simulink model "DT_enviroment_state_machine"  (R2024b)
settings: Solver=FixedStepAuto  StartTime=0.0  StopTime=120  FixedStep=1e-3  RelTol=1e-3
InitFcn:
  | V_bias_cmd=0;
  | enable_cmd=0;
  | mode_cmd=0;
  | P_batt_cmd=0;
libraries: fl_lib x14, nesl_utility x12, batteryecm_lib x2, eeGeneralControl x2, slpidlib x2, simulink x1, spspowerguiLib x1
(part 2 of 2)

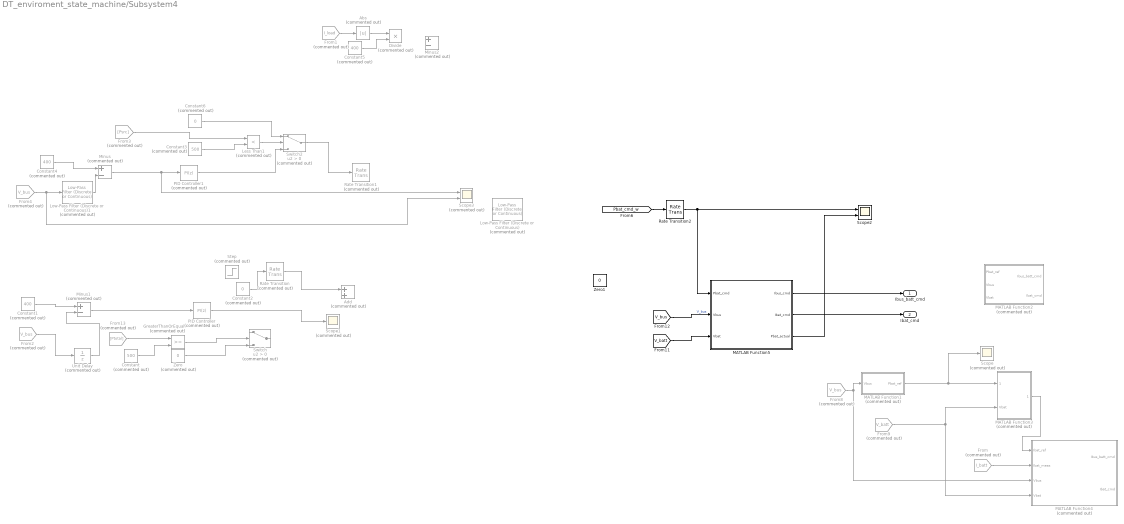
== system DT_enviroment_state_machine/Subsystem4 ==
  Abs : Abs  Commented=on  SaturateOnIntegerOverflow=off
  Add : Sum  Commented=on
  Constant : Constant  Commented=on  Value=500  SampleTime=-1
  Constant1 : Constant  Commented=on  Value=400
  Constant2 : Constant  Commented=on  Value=0  SampleTime=-1
  Constant3 : Constant  Commented=on  Value=500
  Constant4 : Constant  Commented=on  Value=400
  Constant5 : Constant  Commented=on  Value=400
  Constant6 : Constant  Commented=on  Value=0
  Divide : Product  Commented=on  Inputs=**
  From : From  Commented=on  GotoTag=I_batt  TagVisibility=global
  From1 : From  Commented=on  GotoTag=I_load  TagVisibility=global
  From13 : From  Commented=on  GotoTag=Ptotal  TagVisibility=global
  From2 : From  Commented=on  GotoTag=V_bus  TagVisibility=global
  From3 : From  Commented=on  GotoTag=Psrc  TagVisibility=global
  From4 : From  Commented=on  GotoTag=V_bus  TagVisibility=global
  From8 : From  Commented=on  GotoTag=V_bus  TagVisibility=global
  From9 : From  Commented=on  GotoTag=V_batt  TagVisibility=global
  GreaterThanOrEqual : RelationalOperator  Commented=on  OutDataTypeStr=boolean  RndMeth=Simplest  InputSameDT=off
  Less Than1 : RelationalOperator  Commented=on  Operator=<  OutDataTypeStr=boolean  RndMeth=Simplest  InputSameDT=off
  Low-Pass Filter (Discrete or Continuous) : eeGeneralControl/Low-Pass Filter (Discrete or Continuous)  Commented=on  K=1  T=50000/1000  B=inf  A=-inf  init_option=Inherited from block input  x0=0  Ts=-1
  Low-Pass Filter (Discrete or Continuous)1 : eeGeneralControl/Low-Pass Filter (Discrete or Continuous)  Commented=on  K=1  T=50000/1000  B=inf  A=-inf  init_option=Inherited from block input  x0=0  Ts=-1
  MATLAB Function1 : MATLAB Function  Commented=on  TreatAsAtomicUnit=on
  MATLAB Function2 : MATLAB Function  Commented=on  TreatAsAtomicUnit=on
  MATLAB Function3 : MATLAB Function  Commented=on  TreatAsAtomicUnit=on
  MATLAB Function4 : MATLAB Function  Commented=on  TreatAsAtomicUnit=on
  MATLAB Function5 : MATLAB Function  TreatAsAtomicUnit=on
  Minus : Sum  Commented=on  Inputs=+-
  Minus1 : Sum  Commented=on  Inputs=+-
  Minus2 : Sum  Commented=on  Inputs=+-
  PID Controller : slpidlib/PID Controller  Commented=on  Controller=PI  Form=Parallel  TimeDomain=Discrete-time  UseExternalTs=off  SampleTime=-1  IntegratorMethod=Forward Euler  FilterMethod=Forward Euler  ControllerParametersSource=internal  P=0.5  I=1  UseKiTs=off  D=0  UseExternalDerivativeSource=off  N=100  UseFilter=on  TunerSelectOption=Transfer Function Based (PID Tuner App)  InitialConditionSource=internal  InitialConditionForIntegrator=0  InitialConditionForFilter=0  DifferentiatorICPrevScaledInput=0  ExternalReset=none  TrackingMode=off  Kt=1  LimitOutput=off  SatLimitsSource=internal  UpperSaturationLimit=inf  LowerSaturationLimit=-inf  LinearizeAsGain=on  AntiWindupMode=clamping  Kb=1  LimitIntegrator=off  UpperIntegratorSaturationLimit=inf  LowerIntegratorSaturationLimit=-inf  POutMin=[]  POutMax=[]  IOutMin=[]  IOutMax=[]  DOutMin=[]  DOutMax=[]  NOutMin=[]  NOutMax=[]  SumOutMin=[]  SumOutMax=[]  SaturationOutMin=[]  SaturationOutMax=[]  PParamMin=[]  PParamMax=[]  IParamMin=[]  IParamMax=[]  DParamMin=[]  DParamMax=[]  NParamMin=[]  NParamMax=[]  KbParamMin=[]  KbParamMax=[]  KtParamMin=[]  KtParamMax=[]  KbOutMin=[]  KbOutMax=[]  KtOutMin=[]  KtOutMax=[]  IntegratorOutMin=[]  IntegratorOutMax=[]  FilterOutMin=[]  FilterOutMax=[]  SumI1OutMin=[]  SumI1OutMax=[]  SumI2OutMin=[]  SumI2OutMax=[]  SumI3OutMin=[]  SumI3OutMax=[]  SumI4OutMin=[]  SumI4OutMax=[]  SumDOutMin=[]  SumDOutMax=[]  DifferentiatorOutMin=[]  DifferentiatorOutMax=[]  FilterDiffOutCoefMin=[]  FilterDiffOutCoefMax=[]  ReciprocalOutMin=[]  ReciprocalOutMax=[]  SumDenOutMin=[]  SumDenOutMax=[]  SumNumOutMin=[]  SumNumOutMax=[]  DivideOutMin=[]  DivideOutMax=[]  UdiffTsProdOutMin=[]  UdiffTsProdOutMax=[]  NTsProdOutMin=[]  NTsProdOutMax=[]  UintegralTsProdOutMin=[]  UintegralTsProdOutMax=[]  UngainTsProdOutMin=[]  UngainTsProdOutMax=[]  ClampingZeroOutDataTypeStr=Inherit: Inherit via back propagation  ClampingZeroOutMin=[]  ClampingZeroOutMax=[]  FilterDenConstantOutDataTypeStr=Inherit: Inherit via back propagation  FilterDenConstantOutMin=[]  FilterDenConstantOutMax=[]  PCopyOutDataTypeStr=Inherit: Inherit via back propagation  PCopyOutMin=[]  PCopyOutMax=[]  NCopyOutDataTypeStr=Inherit: Inherit via back propagation  NCopyOutMin=[]  NCopyOutMax=[]  IntegratorContinuousStateAttributes=''  IntegratorStateMustResolveToSignalObject=off  IntegratorRTWStateStorageClass=Auto  FilterContinuousStateAttributes=''  FilterStateMustResolveToSignalObject=off  FilterRTWStateStorageClass=Auto  ParallelPVariant=InternalParameters  IdealPVariant=Disabled  IVariant=InternalParameters  DVariant=Disabled  IntegratorVariant=Discrete  SatVariant=Disabled  AWVariant=Passthrough  PCopyVariant=Disabled  TRVariant=Disabled  FdbkBlocksVariant=Forward  IdealPFdbkVariant=Disabled  SatFdbkVariant=Disabled  DerivativeFilterVariant=Disabled  NVariant=Disabled  NCopyVariant=Disabled_SignalSpec  FilterICVariant=Disabled  IntegratorICVariant=InternalICs  ExternalResetVariant=Disabled  TRSumVariant=Passthrough  SumFdbkVariant=Disabled  SumVariant=Sum_PI  TsampFilterVariant=InternalTs  TsampNgainVariant=Passthrough  TsampIntegralVariant=Disabled_SignalSpec  ExternalSaturationOutDataTypeStr=Inherit: Same as second input  DerivativeSourceVariant=Disabled  PreIntVariant=InternalPreInt
  PID Controller1 : slpidlib/PID Controller  Commented=on  Controller=PI  Form=Parallel  TimeDomain=Discrete-time  UseExternalTs=off  SampleTime=-1  IntegratorMethod=Forward Euler  FilterMethod=Forward Euler  ControllerParametersSource=internal  P=0.01  I=1  UseKiTs=off  D=0  UseExternalDerivativeSource=off  N=100  UseFilter=on  TunerSelectOption=Transfer Function Based (PID Tuner App)  InitialConditionSource=internal  InitialConditionForIntegrator=0  InitialConditionForFilter=0  DifferentiatorICPrevScaledInput=0  ExternalReset=none  TrackingMode=off  Kt=1  LimitOutput=on  SatLimitsSource=internal  UpperSaturationLimit=1000  LowerSaturationLimit=-1000  LinearizeAsGain=on  AntiWindupMode=none  Kb=1  LimitIntegrator=off  UpperIntegratorSaturationLimit=inf  LowerIntegratorSaturationLimit=-inf  POutMin=[]  POutMax=[]  IOutMin=[]  IOutMax=[]  DOutMin=[]  DOutMax=[]  NOutMin=[]  NOutMax=[]  SumOutMin=[]  SumOutMax=[]  SaturationOutMin=[]  SaturationOutMax=[]  PParamMin=[]  PParamMax=[]  IParamMin=[]  IParamMax=[]  DParamMin=[]  DParamMax=[]  NParamMin=[]  NParamMax=[]  KbParamMin=[]  KbParamMax=[]  KtParamMin=[]  KtParamMax=[]  KbOutMin=[]  KbOutMax=[]  KtOutMin=[]  KtOutMax=[]  IntegratorOutMin=[]  IntegratorOutMax=[]  FilterOutMin=[]  FilterOutMax=[]  SumI1OutMin=[]  SumI1OutMax=[]  SumI2OutMin=[]  SumI2OutMax=[]  SumI3OutMin=[]  SumI3OutMax=[]  SumI4OutMin=[]  SumI4OutMax=[]  SumDOutMin=[]  SumDOutMax=[]  DifferentiatorOutMin=[]  DifferentiatorOutMax=[]  FilterDiffOutCoefMin=[]  FilterDiffOutCoefMax=[]  ReciprocalOutMin=[]  ReciprocalOutMax=[]  SumDenOutMin=[]  SumDenOutMax=[]  SumNumOutMin=[]  SumNumOutMax=[]  DivideOutMin=[]  DivideOutMax=[]  UdiffTsProdOutMin=[]  UdiffTsProdOutMax=[]  NTsProdOutMin=[]  NTsProdOutMax=[]  UintegralTsProdOutMin=[]  UintegralTsProdOutMax=[]  UngainTsProdOutMin=[]  UngainTsProdOutMax=[]  ClampingZeroOutDataTypeStr=Inherit: Inherit via back propagation  ClampingZeroOutMin=[]  ClampingZeroOutMax=[]  FilterDenConstantOutDataTypeStr=Inherit: Inherit via back propagation  FilterDenConstantOutMin=[]  FilterDenConstantOutMax=[]  PCopyOutDataTypeStr=Inherit: Inherit via back propagation  PCopyOutMin=[]  PCopyOutMax=[]  NCopyOutDataTypeStr=Inherit: Inherit via back propagation  NCopyOutMin=[]  NCopyOutMax=[]  IntegratorContinuousStateAttributes=''  IntegratorStateMustResolveToSignalObject=off  IntegratorRTWStateStorageClass=Auto  FilterContinuousStateAttributes=''  FilterStateMustResolveToSignalObject=off  FilterRTWStateStorageClass=Auto  ParallelPVariant=InternalParameters  IdealPVariant=Disabled  IVariant=InternalParameters  DVariant=Disabled  IntegratorVariant=Discrete  SatVariant=Enabled  AWVariant=Passthrough  PCopyVariant=Disabled  TRVariant=Disabled  FdbkBlocksVariant=Forward  IdealPFdbkVariant=Disabled  SatFdbkVariant=Disabled  DerivativeFilterVariant=Disabled  NVariant=Disabled  NCopyVariant=Disabled_SignalSpec  FilterICVariant=Disabled  IntegratorICVariant=InternalICs  ExternalResetVariant=Disabled  TRSumVariant=Passthrough  SumFdbkVariant=Disabled  SumVariant=Sum_PI  TsampFilterVariant=InternalTs  TsampNgainVariant=Passthrough  TsampIntegralVariant=Disabled_SignalSpec  ExternalSaturationOutDataTypeStr=Inherit: Same as second input  DerivativeSourceVariant=Disabled  PreIntVariant=InternalPreInt
  Rate Transition : RateTransition  Commented=on
  Rate Transition1 : RateTransition  Commented=on
  Rate Transition2 : RateTransition
  Scope : Scope  Commented=on
  Scope1 : Scope  Commented=on
  Scope2 : Scope  NumInputPorts=2
  Scope3 : Scope  Commented=on  NumInputPorts=2
  Step : Step  Commented=on  Time=170  After=-100  SampleTime=0
  Switch : Switch  Commented=on  Criteria=u2 > Threshold  SaturateOnIntegerOverflow=off  InputSameDT=off
  Switch2 : Switch  Commented=on  Criteria=u2 > Threshold  SaturateOnIntegerOverflow=off  InputSameDT=off
  Unit Delay : UnitDelay  Commented=on  SampleTime=-1  HasFrameUpgradeWarning=on
  Zero : Constant  Commented=on  Value=0  OutDataTypeStr=Inherit: Inherit via back propagation  SampleTime=-1
  Zero1 : Constant  Value=0  OutDataTypeStr=Inherit: Inherit via back propagation
  Ibus_batt_cmd : Outport
  Ibat_cmd : Outport  Port=2
  wires:
  From8/1 -> MATLAB Function4/3(Vbus), MATLAB Function1/1(Vbus)
  MATLAB Function5/1(Ibus_cmd) -> Ibus_batt_cmd/1
  MATLAB Function1/1(Pbat_ref) -> Scope/1, MATLAB Function3/1(Pbat_ref)
  From9/1 -> MATLAB Function3/2(Vbat), MATLAB Function4/4(Vbat)
  MATLAB Function3/1(Ibat_ref) -> MATLAB Function4/1(Ibat_ref)
  From/1 -> MATLAB Function4/2(Ibat_meas)
  MATLAB Function5/2(Ibat_cmd) -> Ibat_cmd/1
  [V_bus] -> MATLAB Function5/2(Vbus)  "V_bus"
  [V_batt] -> MATLAB Function5/3(Vbat)
  From13/1 -> GreaterThanOrEqual/1
  Constant/1 -> GreaterThanOrEqual/2
  GreaterThanOrEqual/1 -> Switch/2
  Zero/1 -> Switch/3
  ? -> Switch/1
  Unit Delay/1 -> Minus1/2
  Minus1/1 -> PID Controller/1
  Constant1/1 -> Minus1/1
  PID Controller/1 -> Scope1/1
  Rate Transition/1 -> Add/1
  Constant2/1 -> Rate Transition/1
  From2/1 -> Unit Delay/1
  From1/1 -> Abs/1
  Constant5/1 -> Divide/2
  From3/1 -> Less Than1/1
  Abs/1 -> Divide/1
  Constant3/1 -> Less Than1/2
  Less Than1/1 -> Switch2/2
  Constant6/1 -> Switch2/1
  Switch2/1 -> Rate Transition1/1
  MATLAB Function5/3(Pbat_actual) -> Scope2/2
  PID Controller1/1 -> Switch2/3
  Constant4/1 -> Minus/1
  From4/1 -> Scope3/2, Low-Pass Filter (Discrete or Continuous)1/1
  Minus/1 -> PID Controller1/1, Scope3/1
  Low-Pass Filter (Discrete or Continuous)1/1 -> Minus/2
  Rate Transition2/1 -> MATLAB Function5/1(Pbat_cmd), Scope2/1
  [Pbat_cmd_w] -> Rate Transition2/1

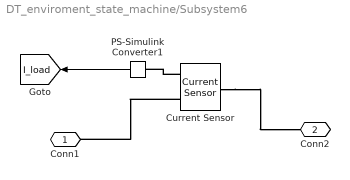
== system DT_enviroment_state_machine/Subsystem6 ==
  Current Sensor : fl_lib/Electrical/Electrical Sensors/Current Sensor
  PS-Simulink Converter1 : nesl_utility/PS-Simulink Converter  PhysicalDomain=network_engine_domain  SubClassName=ps_output  LeftPortType=input  RightPortType=output  PseudoPeriodic=off  Frequencies=[]  VectorFormat=inherit  Unit=inherit  AffineConversion=off
  Conn1 : PMIOPort  Side=Left
  Conn2 : PMIOPort  Port=2  Side=Right
  tag scope: I_load=global
  wires:
  PS-Simulink Converter1/1 -> [I_load]
  connections:
  Current Sensor/RConn1 -- PS-Simulink Converter1/LConn1
  Current Sensor/LConn1 -- Conn2/RConn1
  Current Sensor/RConn2 -- Conn1/RConn1

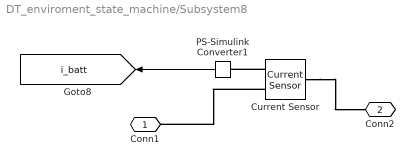
== system DT_enviroment_state_machine/Subsystem8 ==
  Current Sensor : fl_lib/Electrical/Electrical Sensors/Current Sensor
  PS-Simulink Converter1 : nesl_utility/PS-Simulink Converter  PhysicalDomain=network_engine_domain  SubClassName=ps_output  LeftPortType=input  RightPortType=output  PseudoPeriodic=off  Frequencies=[]  VectorFormat=inherit  Unit=inherit  AffineConversion=off
  Conn1 : PMIOPort  Side=Left
  Conn2 : PMIOPort  Port=2  Side=Right
  tag scope: i_batt=global
  wires:
  PS-Simulink Converter1/1 -> [i_batt]
  connections:
  Current Sensor/RConn1 -- PS-Simulink Converter1/LConn1
  Current Sensor/RConn2 -- Conn1/RConn1
  Current Sensor/LConn1 -- Conn2/RConn1

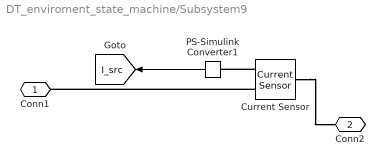
== system DT_enviroment_state_machine/Subsystem9 ==
  Current Sensor : fl_lib/Electrical/Electrical Sensors/Current Sensor
  PS-Simulink Converter1 : nesl_utility/PS-Simulink Converter  PhysicalDomain=network_engine_domain  SubClassName=ps_output  LeftPortType=input  RightPortType=output  PseudoPeriodic=off  Frequencies=[]  VectorFormat=inherit  Unit=inherit  AffineConversion=off
  Conn1 : PMIOPort  Side=Left
  Conn2 : PMIOPort  Port=2  Side=Right
  tag scope: I_src=global
  wires:
  PS-Simulink Converter1/1 -> [I_src]
  connections:
  Current Sensor/RConn1 -- PS-Simulink Converter1/LConn1
  Current Sensor/RConn2 -- Conn1/RConn1
  Current Sensor/LConn1 -- Conn2/RConn1

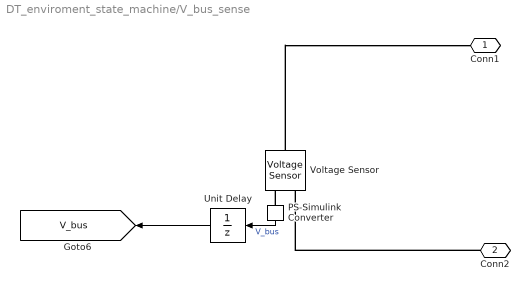
== system DT_enviroment_state_machine/V_bus_sense ==
  PS-Simulink Converter : nesl_utility/PS-Simulink Converter  PhysicalDomain=network_engine_domain  SubClassName=ps_output  LeftPortType=input  RightPortType=output  PseudoPeriodic=off  Frequencies=[]  VectorFormat=inherit  Unit=inherit  AffineConversion=off
  Unit Delay : UnitDelay  InitialCondition=400  SampleTime=-1  HasFrameUpgradeWarning=on
  Voltage Sensor : fl_lib/Electrical/Electrical Sensors/Voltage Sensor
  Conn1 : PMIOPort  Side=Left
  Conn2 : PMIOPort  Port=2  Side=Right
  tag scope: V_bus=global
  wires:
  PS-Simulink Converter/1 -> Unit Delay/1  "V_bus"
  Unit Delay/1 -> [V_bus]
  connections:
  PS-Simulink Converter/LConn1 -- Voltage Sensor/RConn1
  Conn2/RConn1 -- Voltage Sensor/RConn2
  Voltage Sensor/LConn1 -- Conn1/RConn1

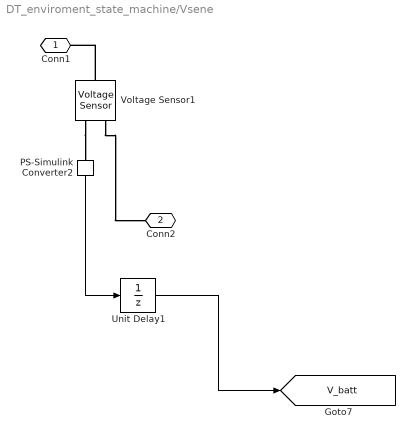
== system DT_enviroment_state_machine/Vsene ==
  PS-Simulink Converter2 : nesl_utility/PS-Simulink Converter  PhysicalDomain=network_engine_domain  SubClassName=ps_output  LeftPortType=input  RightPortType=output  PseudoPeriodic=off  Frequencies=[]  VectorFormat=inherit  Unit=inherit  AffineConversion=off
  Unit Delay1 : UnitDelay  InitialCondition=300  SampleTime=-1  HasFrameUpgradeWarning=on
  Voltage Sensor1 : fl_lib/Electrical/Electrical Sensors/Voltage Sensor
  Conn1 : PMIOPort  Side=Left
  Conn2 : PMIOPort  Port=2  Side=Right
  tag scope: V_batt=global
  wires:
  PS-Simulink Converter2/1 -> Unit Delay1/1
  Unit Delay1/1 -> [V_batt]
  connections:
  Voltage Sensor1/LConn1 -- Conn1/RConn1
  Voltage Sensor1/RConn1 -- PS-Simulink Converter2/LConn1
  Voltage Sensor1/RConn2 -- Conn2/RConn1

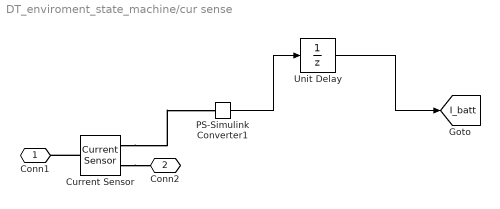
== system DT_enviroment_state_machine/cur sense ==
  Current Sensor : fl_lib/Electrical/Electrical Sensors/Current Sensor
  PS-Simulink Converter1 : nesl_utility/PS-Simulink Converter  PhysicalDomain=network_engine_domain  SubClassName=ps_output  LeftPortType=input  RightPortType=output  PseudoPeriodic=off  Frequencies=[]  VectorFormat=inherit  Unit=inherit  AffineConversion=off
  Unit Delay : UnitDelay  SampleTime=-1  HasFrameUpgradeWarning=on
  Conn1 : PMIOPort  Side=Left
  Conn2 : PMIOPort  Port=2  Side=Right
  tag scope: I_batt=global
  wires:
  PS-Simulink Converter1/1 -> Unit Delay/1
  Unit Delay/1 -> [I_batt]
  connections:
  Current Sensor/RConn1 -- PS-Simulink Converter1/LConn1
  Current Sensor/LConn1 -- Conn1/RConn1
  Current Sensor/RConn2 -- Conn2/RConn1

== matlab function DT_enviroment_state_machine/Subsystem4/MATLAB Function1 ==
  data: Vbus input; Pbat_ref output
% function Pbat_ref = battery_outer_bus_controller(Vbus)
% 
% % Positive Pbat_ref = battery discharges into the bus
% % Negative Pbat_ref = battery charges from the bus
% 
% Vref = 400;
% deadband = 2;
% 
% Pdis_max = 480;   % W, about 12 V * 40 A
% Pchg_max = 300;   % W, about 12 V * 25 A
% 
% Kp = 40;
% 
% err = Vref - Vbus;
% 
% if abs(err) < deadband
%     Pcmd = 0;
% else
%     Pcmd = Kp * err;
% end
% 
% Pbat_ref = min(max(Pcmd, -Pchg_max), Pdis_max);

function Pbat_ref = battery_outer_bus_controller(Vbus)

% Positive Pbat_ref = battery discharges into bus
% Negative Pbat_ref = battery charges from bus

Vref = 400;

Pdis_max = 480;   % W
Pchg_max = 300;   % W

Kp = 80;          % W/V
Ki = 300;         % W/(V*s)

Ts = 1e-3;        % match your controller sample time

persistent integ
if isempty(integ)
    integ = 0;
end

err = Vref - Vbus;

P_unsat = Kp*err + Ki*integ;

Pbat_ref = min(max(P_unsat, -Pchg_max), Pdis_max);

% Anti-windup
if Pbat_ref == P_unsat || ...
   (Pbat_ref == Pdis_max && err < 0) || ...
   (Pbat_ref == -Pchg_max && err > 0)
    integ = integ + err*Ts;
end

== matlab function DT_enviroment_state_machine/Subsystem1/MATLAB Function ==
  data: Isrc output; Vbus input
function Isrc = source_current_command(Vbus)

% 400 V regulated source with 500 W power limit

Vref = 400;
Pmax = 500;

Kp = 0.1;      % A/V
Ki = 5.0;      % A/(V*s)
Ts = 1e-3;     % match your controller sample time

persistent integ
if isempty(integ)
    integ = 0;
end

err = Vref - Vbus;

% Integrate only when bus is below/near reference
integ = integ + err * Ts;

Isrc_cmd = Kp*err + Ki*integ;

% Source cannot absorb current in this simple model
Isrc_cmd = max(Isrc_cmd, 0);

% Power limit
Vsafe = max(abs(Vbus), 100);
Isrc_pmax = Pmax / Vsafe;

% Clamp to power limit and absolute current limit
Iabs_max = 5;
Isrc_unsat = Isrc_cmd;
Isrc = min(Isrc_cmd, Isrc_pmax);
Isrc = min(Isrc, Iabs_max);

% Simple anti-windup: if saturated, back off integrator
if Isrc ~= Isrc_unsat
    integ = integ - err * Ts;
end

== matlab function DT_enviroment_state_machine/Subsystem4/MATLAB Function2 ==
  data: Pbat_ref input; Ibus_batt_cmd output; Vbus input; Vbat input; Ibat_cmd output
function [Ibus_batt_cmd, Ibat_cmd] = battery_power_to_current(Pbat_ref, Vbus, Vbat)

% Positive Pbat_ref = battery discharges into bus
% Positive Ibus_batt_cmd = current injected into bus
% Positive Ibat_cmd = current leaving battery

eta = 1.0;   % ideal for now

Vbus_safe = max(abs(Vbus), 100);
Vbat_safe = max(abs(Vbat), 6);

if Pbat_ref >= 0
    % Discharge: battery power becomes bus power
    Pbus = eta * Pbat_ref;
    Pbat = Pbat_ref;
else
    % Charge: bus supplies battery; ideal case first
    Pbus = Pbat_ref;
    Pbat = Pbat_ref;
end

Ibus_batt_cmd = Pbus / Vbus_safe;
Ibat_cmd = Pbat / Vbat_safe;

% Battery current clamps
Ibat_dis_max = 40;
Ibat_chg_max = 25;

Ibat_cmd = min(max(Ibat_cmd, -Ibat_chg_max), Ibat_dis_max);

% Recompute bus command after current clamp
Pbat_limited = Ibat_cmd * Vbat_safe;
Ibus_batt_cmd = Pbat_limited / Vbus_safe;

== matlab function DT_enviroment_state_machine/Subsystem4/MATLAB Function3 ==
  data: Pbat_ref input; Ibat_ref output; Vbat input
function Ibat_ref = power_to_battery_current(Pbat_ref, Vbat)

% Positive Ibat_ref = battery discharge
% Negative Ibat_ref = battery charge

Vbat_safe = max(abs(Vbat), 6);

Ibat_ref = Pbat_ref / Vbat_safe;

Ibat_ref = min(max(Ibat_ref, -25), 40);

== matlab function DT_enviroment_state_machine/Subsystem4/MATLAB Function4 ==
  data: Ibat_ref input; Ibus_batt_cmd output; Ibat_meas input; Vbus input; Vbat input; Ibat_cmd output
function [Ibus_batt_cmd, Ibat_cmd] = inner_battery_current_controller(Ibat_ref, Ibat_meas, Vbus, Vbat)

% Positive Ibat_ref/Ibat_cmd = battery discharge
% Positive Ibus_batt_cmd = current injected into bus

Kp = 20;       % W/A
Ki = 200;      % W/(A*s)
Ts = 1e-3;

Pdis_max = 480;
Pchg_max = 300;

persistent integ
if isempty(integ)
    integ = 0;
end

err = Ibat_ref - Ibat_meas;

P_unsat = Kp*err + Ki*integ;

Pconv_cmd = min(max(P_unsat, -Pchg_max), Pdis_max);

% Anti-windup
if Pconv_cmd == P_unsat || ...
   (Pconv_cmd == Pdis_max && err < 0) || ...
   (Pconv_cmd == -Pchg_max && err > 0)
    integ = integ + err*Ts;
end

Vbus_safe = max(abs(Vbus), 100);
Vbat_safe = max(abs(Vbat), 6);

Ibus_batt_cmd = Pconv_cmd / Vbus_safe;
Ibat_cmd      = Pconv_cmd / Vbat_safe;

== matlab function DT_enviroment_state_machine/Battery Grid State Machine ==
  data: Vbus_v input; P_batt_ref_w output; soc_pct input; i_load_a input; source_at_limit input; charge_enable input; soc_target_pct input; charge_power_cap_w input; state_code output; charge_headroom_w output; p_load_nominal_w output; voltage_error_v output; vbus_log_v output; soc_log_pct output; source_at_limit_log output
function [P_batt_ref_w, state_code, charge_headroom_w, p_load_nominal_w, voltage_error_v, vbus_log_v, soc_log_pct, source_at_limit_log] = fcn(Vbus_v, soc_pct, i_load_a, source_at_limit, charge_enable, soc_target_pct, charge_power_cap_w)
%#codegen
% Deterministic hybrid battery/grid controller.
% Positive P_batt_ref_w discharges into the DC bus.
% Negative P_batt_ref_w charges the battery.

% State codes.
HOLD = uint8(0);
CHARGE = uint8(1);
BUS_SUPPORT = uint8(2);
SAFE_LOCAL = uint8(3);

% Plant and controller constants kept explicit for auditability.
Ts = 1e-3;
Vnom = 400.0;
Vsupport_enter = 397.0;
Vsupport_exit = 399.0;
Vcharge_abort = 395.0;
Psource_limit = 500.0;
Psource_reserve = 25.0;
Psource_allowed = Psource_limit - Psource_reserve;
Pdis_max = 480.0;
Pchg_max = 300.0;
Kp_v = 5.0;
Ki_v = 2.0;
integral_max_v_s = 15.0;

persistent state integral_v_s
if isempty(state)
    state = HOLD;
    integral_v_s = 0.0;
end

% Use nominal-voltage load power so a voltage sag does not make the
% load appear artificially smaller than the power needed at 400 V.
p_load_nominal_w = Vnom * abs(i_load_a);
charge_headroom_w = max(0.0, Psource_allowed - p_load_nominal_w);
voltage_error_v = max(0.0, Vsupport_exit - Vbus_v);

signals_valid = isfinite(Vbus_v) && isfinite(soc_pct) && isfinite(i_load_a);
hard_fault = ~signals_valid || soc_pct <= 10.0 || soc_pct >= 95.0 || Vbus_v <= 250.0 || Vbus_v >= 500.0;
support_requested = Vbus_v <= Vsupport_enter || source_at_limit >= 0.5 || p_load_nominal_w >= Psource_allowed;
charge_support_requested = Vbus_v <= Vcharge_abort || source_at_limit >= 0.5 || p_load_nominal_w >= Psource_allowed;
support_cleared = Vbus_v >= Vsupport_exit && source_at_limit < 0.5 && p_load_nominal_w <= (Psource_allowed - 10.0);
charge_requested = charge_enable >= 0.5 && soc_pct < (soc_target_pct - 0.1);
charge_entry_possible = charge_requested && charge_headroom_w > 1.0 && Vbus_v >= Vsupport_exit;
charge_continue_possible = charge_requested && charge_headroom_w > 1.0 && Vbus_v > Vcharge_abort && source_at_limit < 0.5;

% Deterministic transition arbitration.  Protection and bus support
% always have more authority than the supervisory charge request.
if hard_fault
    state = SAFE_LOCAL;
else
    switch state
        case SAFE_LOCAL
            state = HOLD;
        case HOLD
            if support_requested
                state = BUS_SUPPORT;
            elseif charge_entry_possible
                state = CHARGE;
            end
        case CHARGE
            if charge_support_requested
                state = BUS_SUPPORT;
            elseif ~charge_continue_possible
                state = HOLD;
            end
        case BUS_SUPPORT
            if support_cleared
                if charge_entry_possible
                    state = CHARGE;
                else
                    state = HOLD;
                end
            end
        otherwise
            state = SAFE_LOCAL;
    end
end

% Continuous command calculation inside the selected state.
switch state
    case CHARGE
        integral_v_s = 0.0;
        requested_charge_w = min(max(abs(charge_power_cap_w), 0.0), Pchg_max);
        P_batt_ref_w = -min(requested_charge_w, charge_headroom_w);
    case BUS_SUPPORT
        p_deficit_w = max(0.0, p_load_nominal_w - Psource_allowed);
        p_unsat_w = p_deficit_w + Kp_v * voltage_error_v + Ki_v * integral_v_s;
        P_batt_ref_w = min(max(p_unsat_w, 0.0), Pdis_max);
        if voltage_error_v > 0.0 && p_unsat_w < Pdis_max
            integral_v_s = min(integral_v_s + voltage_error_v * Ts, integral_max_v_s);
        elseif voltage_error_v <= 0.0
            integral_v_s = max(0.0, integral_v_s - Ts);
        end
    otherwise
        integral_v_s = 0.0;
        P_batt_ref_w = 0.0;
end

state_code = double(state);
vbus_log_v = Vbus_v;
soc_log_pct = soc_pct;
source_at_limit_log = double(source_at_limit >= 0.5);
end

== matlab function DT_enviroment_state_machine/Subsystem4/MATLAB Function5 ==
  data: Pbat_cmd input; Ibus_cmd output; Vbus input; Vbat input; Ibat_cmd output; Pbat_actual output
function [Ibus_cmd, Ibat_cmd, Pbat_actual] = battery_power_interface(Pbat_cmd, Vbus, Vbat)

% Positive Pbat_cmd = battery discharges into DC bus
% Negative Pbat_cmd = battery charges from DC bus

Ts = 1e-3;
tau = 0.01;

eta_dis = 0.95;
eta_chg = 0.95;

Pdis_max = 480;
Pchg_max = 300;

Ibat_dis_max = 40;
Ibat_chg_max = 25;

persistent Pstate
if isempty(Pstate)
    Pstate = 0;
end

% Power limits
Pcmd = min(max(Pbat_cmd, -Pchg_max), Pdis_max);

% Converter response
alpha = Ts/tau;
alpha = min(max(alpha, 0), 1);
Pstate = Pstate + alpha*(Pcmd - Pstate);

Vbus_safe = max(abs(Vbus), 100);
Vbat_safe = max(abs(Vbat), 6);

% Battery-side current
Ibat_cmd = Pstate / Vbat_safe;
Ibat_cmd = min(max(Ibat_cmd, -Ibat_chg_max), Ibat_dis_max);

% Actual battery-side power after current limiting
Pbat_actual = Ibat_cmd * Vbat_safe;

% Bus-side power with efficiency
if Pbat_actual >= 0
    % Discharge: battery power -> bus power
    Pbus = eta_dis * Pbat_actual;
else
    % Charge: bus power -> battery power
    Pbus = Pbat_actual / eta_chg;
end

Ibus_cmd = Pbus / Vbus_safe;
